simulink model "scars_model_lin_test2"  (R2019b)
settings: Solver=FixedStepAuto  StartTime=0.0  StopTime=TFinal*5  FixedStep=0.01  MaxStep=1  MinStep=dT  RelTol=1e-3
model workspace (MAT data in the model file):
  actuators = 0
values from neighbouring files (symbols this model uses):
  initEuler = [0 0 0]    [SCARSSetup.m]    (also in pwsat2_setup.m; scars_setup.m)
  linsys1 = linearize(model,io,op)    [lin_test2_success.m]
undefined symbols (not defined in the file or in its folder): Earth, L_mt, mag_sat, mt_gain, R_mt, WGS84
libraries: scars_library x9, aerolibutil x3, vrlib x2, sharedtransform x2, simulink x1, aerolib6dof2 x1
settings Model: OrderedModelArguments=off  Creator=asmialek  LastModifiedBy=asmialek
settings DataIOCC: SaveFormat=Array  ReturnWorkspaceOutputsName=scars_out

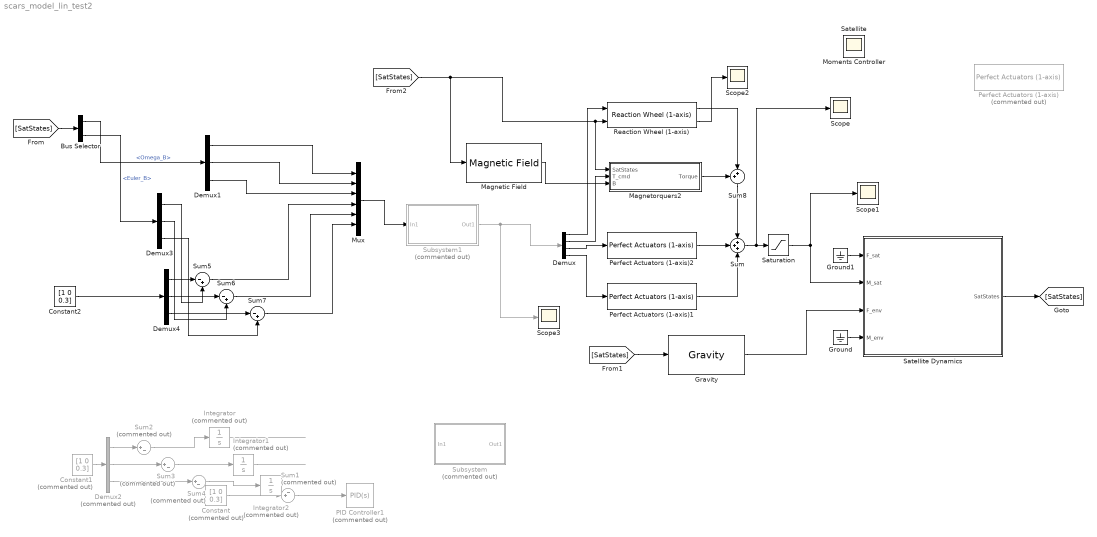
== system scars_model_lin_test2 ==
  Bus Selector : BusSelector  OutputSignals=Omega_B,Euler_B
  Constant : Constant  Commented=on  Value=[1 0 0.3]
  Constant1 : Constant  Commented=on  Value=[1 0 0.3]
  Constant2 : Constant  Value=[1 0 0.3]
  Demux : Demux
  Demux1 : Demux  Outputs=3
  Demux2 : Demux  Commented=on  Outputs=3
  Demux3 : Demux  Outputs=3
  Demux4 : Demux  Outputs=3
  Gravity : scars_library/Environment/Gravity  SystemSampleTime=-1  Latency=0  AutoFrameSizeCalculation=off
  Ground : Ground
  Ground1 : Ground
  Integrator : Integrator  Commented=on
  Integrator1 : Integrator  Commented=on
  Integrator2 : Integrator  Commented=on
  Magnetic Field : scars_library/Environment/Magnetic Field  SystemSampleTime=-1  Latency=0  AutoFrameSizeCalculation=off
  Magnetorquers2 : Subsystem
  Mux : Mux  Inputs=6
  PID Controller1 : simulink/Continuous/PID Controller  Commented=on  Controller=PID  Form=Parallel  TimeDomain=Continuous-time  SampleTime=-1  IntegratorMethod=Forward Euler  FilterMethod=Forward Euler  ControllerParametersSource=internal  P=0.01  I=0.00001  D=0.1  UseFilter=on  N=1  TunerSelectOption=Transfer Function Based (PID Tuner App)  InitialConditionSource=internal  InitialConditionForIntegrator=0  InitialConditionForFilter=0  DifferentiatorICPrevScaledInput=0  ExternalReset=none  TrackingMode=off  Kt=1  LimitOutput=off  UpperSaturationLimit=inf  LowerSaturationLimit=-inf  LinearizeAsGain=on  AntiWindupMode=none  Kb=1  POutMin=[]  POutMax=[]  IOutMin=[]  IOutMax=[]  DOutMin=[]  DOutMax=[]  NOutMin=[]  NOutMax=[]  SumOutMin=[]  SumOutMax=[]  SaturationOutMin=[]  SaturationOutMax=[]  PParamMin=[]  PParamMax=[]  IParamMin=[]  IParamMax=[]  DParamMin=[]  DParamMax=[]  NParamMin=[]  NParamMax=[]  KbParamMin=[]  KbParamMax=[]  KtParamMin=[]  KtParamMax=[]  KbOutMin=[]  KbOutMax=[]  KtOutMin=[]  KtOutMax=[]  IntegratorOutMin=[]  IntegratorOutMax=[]  FilterOutMin=[]  FilterOutMax=[]  SumI1OutMin=[]  SumI1OutMax=[]  SumI2OutMin=[]  SumI2OutMax=[]  SumI3OutMin=[]  SumI3OutMax=[]  SumI4OutMin=[]  SumI4OutMax=[]  SumDOutMin=[]  SumDOutMax=[]  DifferentiatorOutMin=[]  DifferentiatorOutMax=[]  FilterDiffOutCoefMin=[]  FilterDiffOutCoefMax=[]  ReciprocalOutMin=[]  ReciprocalOutMax=[]  SumDenOutMin=[]  SumDenOutMax=[]  SumNumOutMin=[]  SumNumOutMax=[]  DivideOutMin=[]  DivideOutMax=[]  IntegratorContinuousStateAttributes=''  IntegratorStateMustResolveToSignalObject=off  IntegratorRTWStateStorageClass=Auto  FilterContinuousStateAttributes='position'  FilterStateIdentifier=FilterPID  FilterStateMustResolveToSignalObject=on  FilterRTWStateStorageClass=Auto  ParallelPVariant=InternalParameters  IdealPVariant=Disabled  IVariant=InternalParameters  DVariant=InternalParameters  IntegratorVariant=Continuous  SatVariant=Disabled  AWVariant=Passthrough  PCopyVariant=Disabled  TRVariant=Disabled  FdbkBlocksVariant=Forward  IdealPFdbkVariant=Disabled  SatFdbkVariant=Disabled  DerivativeFilterVariant=ContFilter  NVariant=InternalParameters  NCopyVariant=Disabled  FilterICVariant=InternalICsFilter  IntegratorICVariant=InternalICs  ExternalResetVariant=Disabled  TRSumVariant=Passthrough  SumFdbkVariant=Disabled  SumVariant=Sum_PID
  Perfect Actuators (1-axis) : scars_library/Actuators/Perfect Actuators (1-axis)  Commented=on  axis_switch=X  k=1
  Perfect Actuators (1-axis)1 : scars_library/Actuators/Perfect Actuators (1-axis)  axis_switch=Z  k=1
  Perfect Actuators (1-axis)2 : scars_library/Actuators/Perfect Actuators (1-axis)  axis_switch=Y  k=1
  Reaction Wheel (1-axis) : scars_library/Actuators/Reaction Wheel (1-axis)  axis_switch=X  N=25e-3  R=0.1  J=1  c=0.0001
  Satellite Dynamics : Subsystem  AncestorBlock=scars_library/Advanced/Satellite Dynamics
  Saturation : Saturate  UpperLimit=1  LowerLimit=-1
  Scope{,1..3} (4 alike) : Scope
  Subsystem : Subsystem  Commented=on  mask{A=[[linsys1.A; zeros(3, 3) diag([1 1 1])], zeros(9,3)], B=[linsys1.B; zeros(3,3)], Q=diag([100 100 100 0.1 0.1 0.1 200 200 200]), R=diag([ 1 1 1 ])}
      mask init:
      | K = lqr(A, B, Q, R)
  Subsystem1 : Subsystem  Commented=on  mask{A=linsys1.A(12:17,12:17), B=linsys1.B(12:17,1:3), Q=diag([1000 1000 1000 10 10 10]/10), R=diag([ 1 1 1 ])}
      mask init:
      | K = lqr(A, B, Q, R)
  Sum : Sum  Inputs=+++
  Sum1 : Sum  Commented=on  Inputs=-+|
  Sum2 : Sum  Commented=on  Inputs=|+-
  Sum3 : Sum  Commented=on  Inputs=|+-
  Sum4 : Sum  Commented=on  Inputs=|+-
  Sum5 : Sum  Inputs=|-+
  Sum6 : Sum  Inputs=|-+
  Sum7 : Sum  Inputs=|-+
  Sum8 : Sum  Inputs=++|
  Moments Controller : Scope
  Satellite : Scope
  wires:
  Gravity/1 -> Satellite Dynamics/3(F_env)
  Ground/1 -> Satellite Dynamics/4(M_env)
  Ground1/1 -> Satellite Dynamics/1(F_sat)
  Perfect Actuators (1-axis)2/1 -> Sum/2
  Perfect Actuators (1-axis)1/1 -> Sum/3
  Sum/1 -> Scope/1, Saturation/1
  Sum1/1 -> PID Controller1/1
  Satellite Dynamics/1(SatStates) -> [SatStates]
  [SatStates] -> Bus Selector/1
  Constant/1 -> Sum1/2
  Demux/1 -> Reaction Wheel (1-axis)/1
  [SatStates] -> Gravity/1
  Saturation/1 -> Scope1/1, Satellite Dynamics/2(M_sat)
  Demux1/3 -> Mux/3
  Demux1/2 -> Mux/2
  Demux1/1 -> Mux/1
  Subsystem1/1(Out1) -> Scope3/1, Demux/1
  Mux/1 -> Subsystem1/1(In1)
  Bus Selector/1 -> Demux1/1  "<Omega_B>"
  Bus Selector/2 -> Demux3/1  "<Euler_B>"
  Sum4/1 -> Integrator2/1
  Demux2/1 -> Sum2/1
  Constant1/1 -> Demux2/1
  ? -> Sum4/2
  Demux2/2 -> Sum3/1
  Demux2/3 -> Sum4/1
  Sum3/1 -> Integrator1/1
  Sum2/1 -> Integrator/1
  ? -> Sum2/2
  ? -> Sum3/2
  Integrator/1 -> ?
  Integrator1/1 -> ?
  Demux4/1 -> Sum5/1
  Demux4/2 -> Sum6/1
  Demux4/3 -> Sum7/1
  Constant2/1 -> Demux4/1
  Demux3/1 -> Sum5/2
  Demux3/2 -> Sum6/2
  Demux3/3 -> Sum7/2
  Sum5/1 -> Mux/4
  Sum6/1 -> Mux/5
  Sum7/1 -> Mux/6
  [SatStates] -> Magnetorquers2/1(SatStates), Reaction Wheel (1-axis)/2, Magnetic Field/1
  Reaction Wheel (1-axis)/2 -> Scope2/1
  Magnetorquers2/1(Torque) -> Sum8/1
  Reaction Wheel (1-axis)/1 -> Sum8/2
  Sum8/1 -> Sum/1
  Magnetic Field/1 -> Magnetorquers2/3(B)
  Demux/4 -> Perfect Actuators (1-axis)1/1
  Demux/3 -> Perfect Actuators (1-axis)2/1
  Demux/2 -> Magnetorquers2/2(T_cmd)

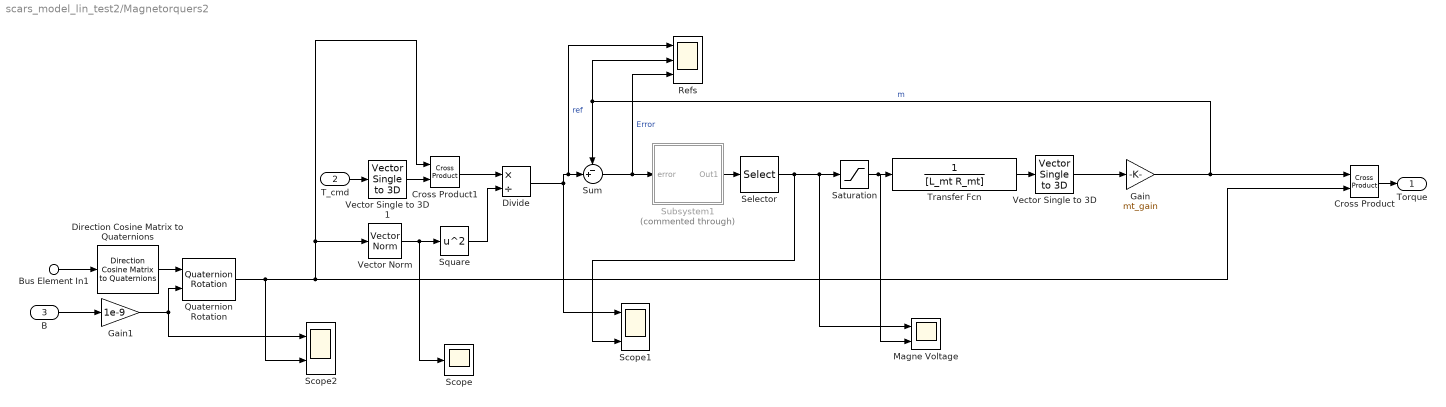
== system scars_model_lin_test2/Magnetorquers2 ==
  Bus Element In1 : Inport  PortName=SatStates  Element=NED2Body
  T_cmd : Inport  Port=2
  B : Inport  Port=3
  Cross Product : vrlib/Utilities/Cross Product
      settings: SourceProductName=Simulink
  Cross Product1 : vrlib/Utilities/Cross Product
      settings: SourceProductName=Simulink
  Direction Cosine Matrix to Quaternions : sharedtransform/Direction Cosine Matrix  to Quaternions  aMode=0  action=None  tolerance=eps(2)
      settings: SourceProductName=Aerospace Blockset  SourceProductBaseCode=AE
  Divide : Product  Inputs=*/
  Gain : Gain  Gain=mt_gain
  Gain1 : Gain  Gain=1e-9
  Magne Voltage : Scope  NumInputPorts=2
  Quaternion Rotation : aerolibutil/Quaternion Rotation
  Refs : Scope  NumInputPorts=3
  Saturation : Saturate  UpperLimit=mag_sat  LowerLimit=-mag_sat
  Scope : Scope
  Scope1 : Scope  NumInputPorts=3
  Scope2 : Scope  NumInputPorts=2
  Selector : Selector  InputPortWidth=3  IndexOptions=Index vector (dialog)  Indices=1  OutputSizes=1
  Square : Math  Operator=square  SignedPower=off  SaturateOnIntegerOverflow=on
  Subsystem1 : Subsystem  Commented=through
  Sum : Sum  Inputs=-+|
  Transfer Fcn : TransferFcn  Denominator=[L_mt R_mt]
  Vector Norm : scars_library/Vector Norm  SystemSampleTime=-1  Latency=0  AutoFrameSizeCalculation=off
  "Vector Single to 3D " : scars_library/Actuators/Vector Single to 3D   axis_switch=1
  Vector Single to 3D 1 : scars_library/Actuators/Vector Single to 3D   axis_switch=1
  Torque : Outport
  wires:
  Divide/1 -> Sum/2, Refs/1, Scope1/1  "ref"
  Subsystem1/1(Out1) -> Selector/1
  Cross Product1/1 -> Divide/1
  Sum/1 -> Subsystem1/1(error), Refs/3  "Error"
  Quaternion Rotation/1 -> Scope2/2, Cross Product/2, Cross Product1/1, Vector Norm/1
  Square/1 -> Divide/2
  Vector Norm/1 -> Scope/1, Square/1
  Saturation/1 -> Magne Voltage/2, Transfer Fcn/1
  B/1 -> Gain1/1
  Bus Element In1/1 -> Direction Cosine Matrix to Quaternions/1
  Direction Cosine Matrix to Quaternions/1 -> Quaternion Rotation/1
  Cross Product/1 -> Torque/1
  Gain/1 -> Sum/1, Refs/2, Cross Product/1  "m"
  Gain1/1 -> Scope2/1, Quaternion Rotation/2
  Transfer Fcn/1 -> "Vector Single to 3D "/1
  "Vector Single to 3D "/1 -> Gain/1
  T_cmd/1 -> Vector Single to 3D 1/1
  Vector Single to 3D 1/1 -> Cross Product1/2
  Selector/1 -> Scope1/3, Saturation/1, Magne Voltage/1

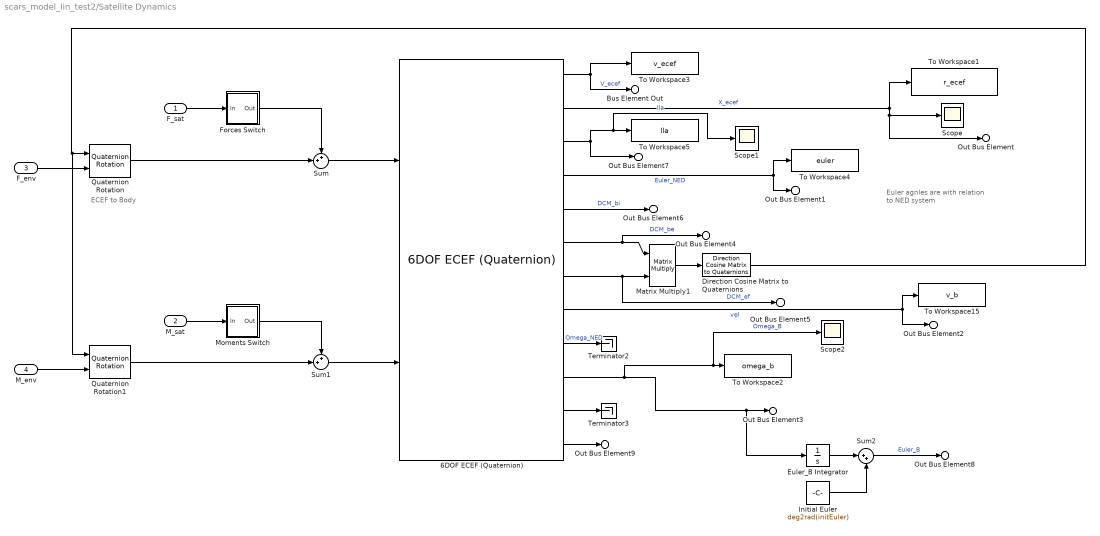
== system scars_model_lin_test2/Satellite Dynamics ==
  note: ECEF to Body
  note: Euler agnles are with relation to NED system
  F_sat : Inport
  M_sat : Inport  Port=2
  F_env : Inport  Port=3
  M_env : Inport  Port=4
  6DOF ECEF (Quaternion) : aerolib6dof2/6DOF ECEF (Quaternion)  units=Metric (MKS)  mtype=Fixed  xg_0=r_lla  Vm_0=v_b  eul_0=deg2rad(initEuler)  pm_0=initEulerRates  mass_0=mass  mass_e=0.5  mass_f=2.0  inertia=eye(3)  inertia_e=eye(3)  inertia_f=2*eye(3)  vre_flag=on  abi_flag=off  ptype=Earth (WGS84)  R=6378137  F=1/298.257223563  w_E=7292115e-11  angle_in=Internal  LG0=0  quat_statename=''  pm_statename=''  Vm_statename=''  posECEF_statename=''  posECI_statename=''  LG_statename=''  mass_statename=''
      settings: SourceProductName=Aerospace Blockset  SourceProductBaseCode=AE
  Direction Cosine Matrix to Quaternions : sharedtransform/Direction Cosine Matrix  to Quaternions  aMode=0  action=None  tolerance=eps(2)
      settings: SourceProductName=Aerospace Blockset  SourceProductBaseCode=AE
  Euler_B Integrator : Integrator
  Forces Switch : Subsystem
  Initial Euler : Constant  Value=deg2rad(initEuler)
  Matrix Multiply1 : Product  Multiplication=Matrix(*)
  Moments Switch : Subsystem
  Quaternion Rotation : aerolibutil/Quaternion Rotation
  Quaternion Rotation1 : aerolibutil/Quaternion Rotation
  Scope : Scope
  Scope1 : Scope
  Scope2 : Scope
  Sum : Sum  Inputs=++|
  Sum1 : Sum  Inputs=++|
  Sum2 : Sum  Inputs=|++
  Terminator2 : Terminator
  Terminator3 : Terminator
  To Workspace1 : ToWorkspace  VariableName=r_ecef  SampleTime=-1
  To Workspace15 : ToWorkspace  VariableName=v_b  SampleTime=-1
      settings: Save2DSignal=2-D array (concatenate along first dimension)
  To Workspace2 : ToWorkspace  VariableName=omega_b  SampleTime=-1
      settings: Save2DSignal=2-D array (concatenate along first dimension)
  To Workspace3 : ToWorkspace  VariableName=v_ecef  SampleTime=-1
      settings: Save2DSignal=2-D array (concatenate along first dimension)
  To Workspace4 : ToWorkspace  VariableName=euler  SampleTime=-1
      settings: Save2DSignal=2-D array (concatenate along first dimension)
  To Workspace5 : ToWorkspace  VariableName=lla  SampleTime=-1
      settings: Save2DSignal=2-D array (concatenate along first dimension)
  Bus Element Out : Outport  PortName=SatStates  Element=V_ecef
  Out Bus Element : Outport  PortName=SatStates  Element=X_ecef
  Out Bus Element1 : Outport  PortName=SatStates  Element=Euler_NED
  Out Bus Element2 : Outport  PortName=SatStates  Element=V_B
  Out Bus Element3 : Outport  PortName=SatStates  Element=Omega_B
  Out Bus Element6 : Outport  PortName=SatStates  Element=ECI2Body
  Out Bus Element4 : Outport  PortName=SatStates  Element=NED2Body
  Out Bus Element5 : Outport  PortName=SatStates  Element=ECEF2NED
  Out Bus Element7 : Outport  PortName=SatStates  Element=lla
  Out Bus Element8 : Outport  PortName=SatStates  Element=Euler_B
  Out Bus Element9 : Outport  PortName=SatStates  Element=A_B
  wires:
  M_env/1 -> Quaternion Rotation1/2
  Sum2/1 -> Out Bus Element8/1  "Euler_B"
  Euler_B Integrator/1 -> Sum2/1
  Initial Euler/1 -> Sum2/2
  Sum/1 -> 6DOF ECEF (Quaternion)/1
  6DOF ECEF (Quaternion)/3 -> To Workspace5/1, Scope1/1, Out Bus Element7/1  "lla"
  6DOF ECEF (Quaternion)/12 -> Out Bus Element9/1
  6DOF ECEF (Quaternion)/11 -> Terminator3/1
  6DOF ECEF (Quaternion)/9 -> Terminator2/1  "Omega_NED"
  6DOF ECEF (Quaternion)/5 -> Out Bus Element6/1  "DCM_bi"
  Moments Switch/1(Out) -> Sum1/1
  M_sat/1 -> Moments Switch/1(In)
  Forces Switch/1(Out) -> Sum/1
  Direction Cosine Matrix to Quaternions/1 -> Quaternion Rotation/1, Quaternion Rotation1/1
  F_env/1 -> Quaternion Rotation/2
  Quaternion Rotation/1 -> Sum/2
  F_sat/1 -> Forces Switch/1(In)
  Matrix Multiply1/1 -> Direction Cosine Matrix to Quaternions/1
  Sum1/1 -> 6DOF ECEF (Quaternion)/2
  Quaternion Rotation1/1 -> Sum1/2
  6DOF ECEF (Quaternion)/10 -> Out Bus Element3/1, Euler_B Integrator/1, To Workspace2/1, Scope2/1  "Omega_B"
  6DOF ECEF (Quaternion)/4 -> To Workspace4/1, Out Bus Element1/1  "Euler_NED"
  6DOF ECEF (Quaternion)/7 -> Matrix Multiply1/2, Out Bus Element5/1  "DCM_ef"
  6DOF ECEF (Quaternion)/6 -> Matrix Multiply1/1, Out Bus Element4/1  "DCM_be"
  6DOF ECEF (Quaternion)/2 -> To Workspace1/1, Out Bus Element/1, Scope/1  "X_ecef"
  6DOF ECEF (Quaternion)/8 -> Out Bus Element2/1, To Workspace15/1  "vel"
  6DOF ECEF (Quaternion)/1 -> Bus Element Out/1, To Workspace3/1  "V_ecef"

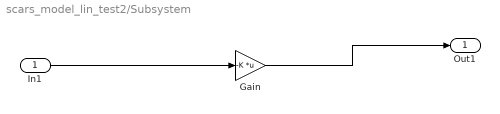
== system scars_model_lin_test2/Subsystem ==
  In1 : Inport
  Gain : Gain  Gain=-K  Multiplication=Matrix(K*u)
  Out1 : Outport
  wires:
  In1/1 -> Gain/1
  Gain/1 -> Out1/1

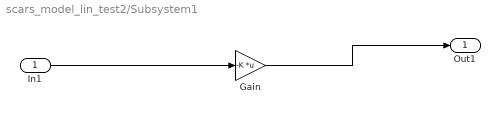
== system scars_model_lin_test2/Subsystem1 ==
  In1 : Inport
  Gain : Gain  Gain=-K  Multiplication=Matrix(K*u)
  Out1 : Outport
  wires:
  Gain/1 -> Out1/1
  In1/1 -> Gain/1

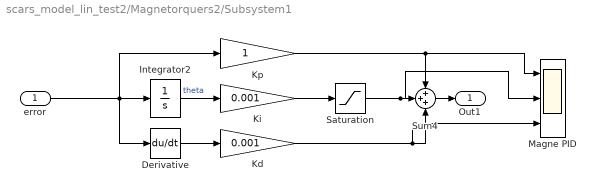
== system scars_model_lin_test2/Magnetorquers2/Subsystem1 ==
  error : Inport
  Derivative : Derivative
  Integrator2 : Integrator
  Kd : Gain  Gain=0.001
  Ki : Gain  Gain=0.001
  Kp : Gain
  Magne PID : Scope  NumInputPorts=3
  Saturation : Saturate  UpperLimit=1  LowerLimit=-1
  Sum4 : Sum  Inputs=+++
  Out1 : Outport
  wires:
  Saturation/1 -> Sum4/2, Magne PID/2
  Kd/1 -> Sum4/3, Magne PID/3
  Derivative/1 -> Kd/1
  Ki/1 -> Saturation/1
  Kp/1 -> Sum4/1, Magne PID/1
  Sum4/1 -> Out1/1
  Integrator2/1 -> Ki/1  "theta"
  error/1 -> Integrator2/1, Derivative/1, Kp/1

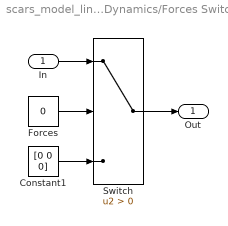
== system scars_model_lin_test2/Satellite Dynamics/Forces Switch ==
  In : Inport
  Constant1 : Constant  Value=[0 0 0]
  Forces : Constant  Value=0
  Switch : Switch  Criteria=u2 > Threshold
  Out : Outport
  wires:
  In/1 -> Switch/1
  Switch/1 -> Out/1
  Forces/1 -> Switch/2
  Constant1/1 -> Switch/3

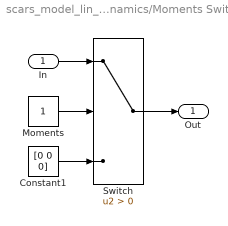
== system scars_model_lin_test2/Satellite Dynamics/Moments Switch ==
  In : Inport
  Constant1 : Constant  Value=[0 0 0]
  Moments : Constant
  Switch : Switch  Criteria=u2 > Threshold
  Out : Outport
  wires:
  Moments/1 -> Switch/2
  Switch/1 -> Out/1
  Constant1/1 -> Switch/3
  In/1 -> Switch/1
